simulink model "test_1"  (Simulink 8.9)
settings: Solver=FixedStepAuto  StartTime=0.0  StopTime=inf  FixedStep=0.1  RelTol=1e-3  EnableMultiTasking=on
libraries: Solver_SF x1, sldrtlib x1, simulink x1
settings Model: Creator=anan  ModifiedByFormat=an  LastModifiedBy=an
settings DataIOCC: ExternalInput=[t, input_1]  SignalLoggingSaveFormat=Dataset
settings OptimizationCC: ExpressionDepthLimit=2147483647
settings DebuggingCC: SolverPrmCheckMsg=warning

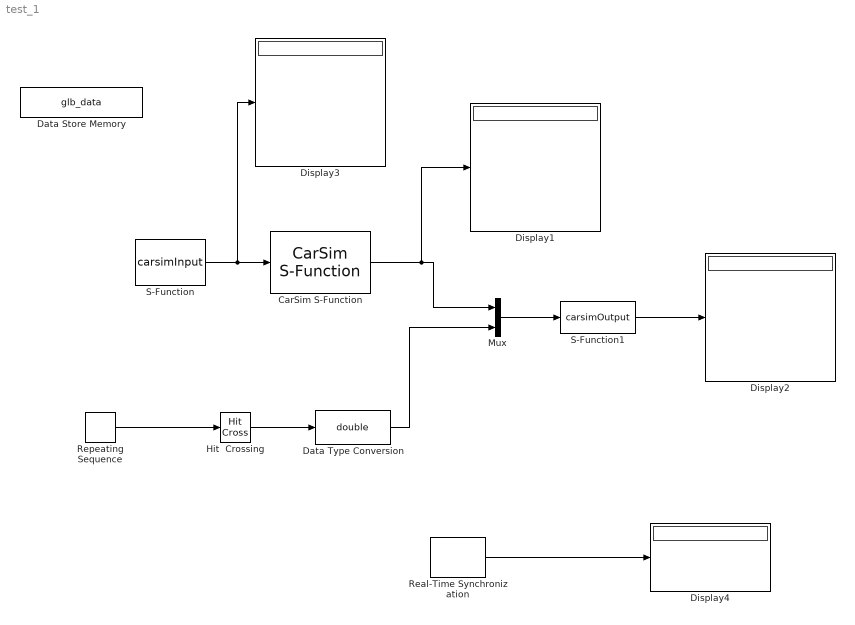
== system test_1 ==
  CarSim S-Function : Solver_SF/CarSim S-Function  Priority=1  VehicleCode=i_s  SIMFILE=simfile.sim
  Data Store Memory : DataStoreMemory  DataStoreName=glb_data  ReadBeforeWriteMsg=warning  WriteAfterWriteMsg=warning  WriteAfterReadMsg=warning  ShowAdditionalParam=off  OutDataTypeStr=double
  Data Type Conversion : DataTypeConversion  OutDataTypeStr=double
  Display{1..4} (4 alike) : Display
      settings: Decimation=2
  Hit  Crossing : HitCross  HitCrossingOffset=0.5  HitCrossingDirection=rising
  Mux : Mux  Inputs=2
  Real-Time Synchronization : sldrtlib/Real-Time Synchronization  SampleTime=0.1  MaxMissedTicks=100000  ShowMissedTicks=on  YieldWhenWaiting=off
  Repeating Sequence : simulink/Sources/Repeating Sequence  rep_seq_t=[0 0.03]  rep_seq_y=[0 2]
  S-Function : S-Function  FunctionName=carsimInput  SFunctionDeploymentMode=off  EnableBusSupport=off
  S-Function1 : S-Function  FunctionName=carsimOutput  SFunctionDeploymentMode=off  EnableBusSupport=off
  wires:
  S-Function/1 -> Display3/1, CarSim S-Function/1
  S-Function1/1 -> Display2/1
  CarSim S-Function/1 -> Display1/1, Mux/1
  Data Type Conversion/1 -> Mux/2
  Hit  Crossing/1 -> Data Type Conversion/1
  Repeating Sequence/1 -> Hit  Crossing/1
  Real-Time Synchronization/1 -> Display4/1
  Mux/1 -> S-Function1/1
